simulink model "cal_hist_bin"  (R2015a)
settings: Solver=ode45  StartTime=0.0  StopTime=10.0  RelTol=1e-3
InitFcn:
  | %% DSPBuilder Start
  | alt_dspbuilder_update_model(bdroot)
  | %% DSPBuilder End
libraries: allblocks_alteradspbuilder2 x705
(part 1 of 9)
settings Model: Creator=ASUS  LastModifiedBy=ASUS

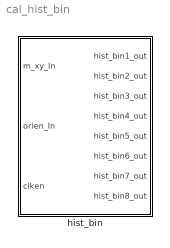
== system cal_hist_bin ==
  hist_bin : Subsystem

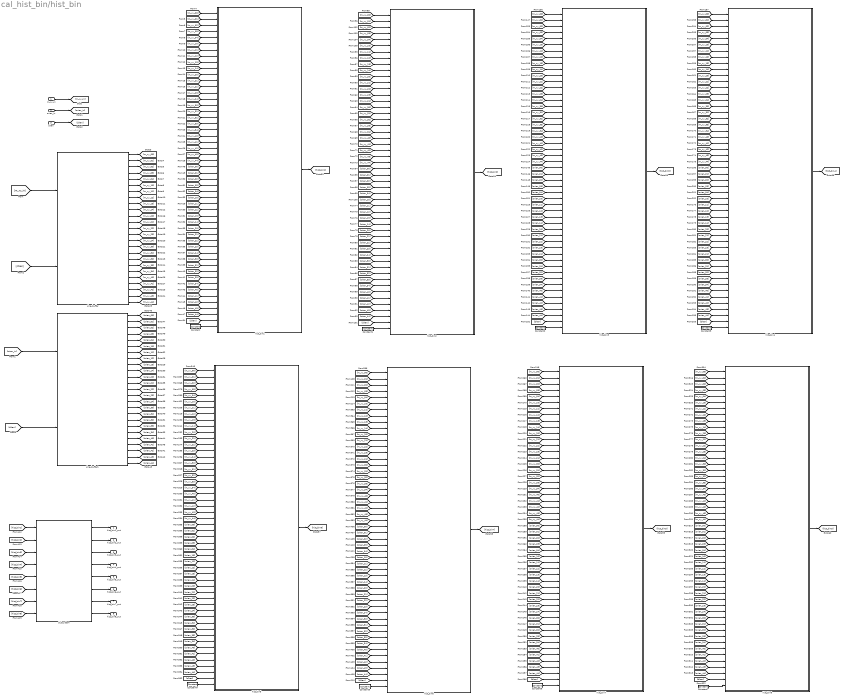
== system cal_hist_bin/hist_bin ==
  m_xy_In : Inport
  orien_In : Inport  Port=2
  clken : Inport  Port=3
  Constant : allblocks_alteradspbuilder2/Constant  mask_cst=1  BusType=Unsigned Integer  bwl=8  bwr=0  roundMode=Truncate  satMode=Wrap  SpecifyClock=off  allowFloatingPointOverride=on  logOutputs=off  logFile=C:\Users\ASUS\Desktop\sift_fpga_final\Octave_1\GradOrien\tb_Untitled1\Untitled1_hist%5Fbin_Constant.fixedpointlog
  Constant1 : allblocks_alteradspbuilder2/Constant  mask_cst=2  BusType=Unsigned Integer  bwl=8  bwr=0  roundMode=Truncate  satMode=Wrap  SpecifyClock=off  allowFloatingPointOverride=on  logOutputs=off  logFile=C:\Users\ASUS\Desktop\sift_fpga_final\Octave_1\GradOrien\tb_Untitled1\Untitled1_hist%5Fbin_Constant1.fixedpointlog
  Constant2 : allblocks_alteradspbuilder2/Constant  mask_cst=3  BusType=Unsigned Integer  bwl=8  bwr=0  roundMode=Truncate  satMode=Wrap  SpecifyClock=off  allowFloatingPointOverride=on  logOutputs=off  logFile=C:\Users\ASUS\Desktop\sift_fpga_final\Octave_1\GradOrien\tb_Untitled1\Untitled1_hist%5Fbin_Constant2.fixedpointlog
  Constant3 : allblocks_alteradspbuilder2/Constant  mask_cst=4  BusType=Unsigned Integer  bwl=8  bwr=0  roundMode=Truncate  satMode=Wrap  SpecifyClock=off  allowFloatingPointOverride=on  logOutputs=off  logFile=C:\Users\ASUS\Desktop\sift_fpga_final\Octave_1\GradOrien\tb_Untitled1\Untitled1_hist%5Fbin_Constant3.fixedpointlog
  Constant4 : allblocks_alteradspbuilder2/Constant  mask_cst=8  BusType=Unsigned Integer  bwl=8  bwr=0  roundMode=Truncate  satMode=Wrap  SpecifyClock=off  allowFloatingPointOverride=on  logOutputs=off  logFile=C:\Users\ASUS\Desktop\sift_fpga_final\Octave_1\GradOrien\tb_Untitled1\Untitled1_hist%5Fbin_Constant4.fixedpointlog
  Constant5 : allblocks_alteradspbuilder2/Constant  mask_cst=7  BusType=Unsigned Integer  bwl=8  bwr=0  roundMode=Truncate  satMode=Wrap  SpecifyClock=off  allowFloatingPointOverride=on  logOutputs=off  logFile=C:\Users\ASUS\Desktop\sift_fpga_final\Octave_1\GradOrien\tb_Untitled1\Untitled1_hist%5Fbin_Constant5.fixedpointlog
  Constant6 : allblocks_alteradspbuilder2/Constant  mask_cst=6  BusType=Unsigned Integer  bwl=8  bwr=0  roundMode=Truncate  satMode=Wrap  SpecifyClock=off  allowFloatingPointOverride=on  logOutputs=off  logFile=C:\Users\ASUS\Desktop\sift_fpga_final\Octave_1\GradOrien\tb_Untitled1\Untitled1_hist%5Fbin_Constant6.fixedpointlog
  Constant7 : allblocks_alteradspbuilder2/Constant  mask_cst=5  BusType=Unsigned Integer  bwl=8  bwr=0  roundMode=Truncate  satMode=Wrap  SpecifyClock=off  allowFloatingPointOverride=on  logOutputs=off  logFile=C:\Users\ASUS\Desktop\sift_fpga_final\Octave_1\GradOrien\tb_Untitled1\Untitled1_hist%5Fbin_Constant7.fixedpointlog
  Line_buffer : Subsystem
  Line_buffer1 : Subsystem
  Subsystem : Subsystem
  hist_bin1 : Subsystem
  hist_bin2 : Subsystem
  hist_bin3 : Subsystem
  hist_bin4 : Subsystem
  hist_bin5 : Subsystem
  hist_bin6 : Subsystem
  hist_bin7 : Subsystem
  hist_bin8 : Subsystem
  hist_bin1_out : Outport
  hist_bin2_out : Outport  Port=2
  hist_bin3_out : Outport  Port=3
  hist_bin4_out : Outport  Port=4
  hist_bin5_out : Outport  Port=5
  hist_bin6_out : Outport  Port=6
  hist_bin7_out : Outport  Port=7
  hist_bin8_out : Outport  Port=8
  wires:
  [hist_bin7] -> Subsystem/7(hist_in_bin7)
  [m_xy_in] -> Line_buffer/1(dataIn)
  [clken] -> Line_buffer/2(clken)
  [clken] -> Line_buffer1/2(clken)
  [orien_in] -> Line_buffer1/1(dataIn)
  clken/1 -> [clken]
  Line_buffer1/21(Out40) -> [orien_40]
  Line_buffer1/19(Out33) -> [orien_33]
  Line_buffer1/8(Out12) -> [orien_12]
  Line_buffer1/14(Out23) -> [orien_23]
  Line_buffer1/18(Out32) -> [orien_32]
  Line_buffer1/20(Out34) -> [orien_34]
  Line_buffer1/2(Out01) -> [orien_01]
  Line_buffer1/7(Out11) -> [orien_11]
  Line_buffer1/11(Out20) -> [orien_20]
  Line_buffer1/13(Out22) -> [orien_22]
  Line_buffer1/17(Out31) -> [orien_31]
  Line_buffer1/25(Out44) -> [orien_44]
  Line_buffer1/3(Out02) -> [orien_02]
  Line_buffer1/5(Out04) -> [orien_04]
  Line_buffer1/23(Out42) -> [orien_42]
  Line_buffer1/24(Out43) -> [orien_43]
  Line_buffer1/6(Out10) -> [orien_10]
  Line_buffer1/1(Out00) -> [orien_00]
  Line_buffer1/22(Out41) -> [orien_41]
  Line_buffer1/15(Out24) -> [orien_24]
  Line_buffer1/4(Out03) -> [orien_03]
  Line_buffer1/9(Out13) -> [orien_13]
  Line_buffer1/10(Out14) -> [orien_14]
  Line_buffer1/12(Out21) -> [orien_21]
  Line_buffer1/16(Out30) -> [orien_30]
  Line_buffer/24(Out43) -> [m_xy_43]
  Line_buffer/21(Out40) -> [m_xy_40]
  Line_buffer/23(Out42) -> [m_xy_42]
  Line_buffer/22(Out41) -> [m_xy_41]
  Line_buffer/25(Out44) -> [m_xy_44]
  Line_buffer/12(Out21) -> [m_xy_21]
  Line_buffer/15(Out24) -> [m_xy_24]
  Line_buffer/19(Out33) -> [m_xy_33]
  Line_buffer/18(Out32) -> [m_xy_32]
  Line_buffer/13(Out22) -> [m_xy_22]
  Line_buffer/11(Out20) -> [m_xy_20]
  Line_buffer/16(Out30) -> [m_xy_30]
  Line_buffer/14(Out23) -> [m_xy_23]
  Line_buffer/17(Out31) -> [m_xy_31]
  Line_buffer/20(Out34) -> [m_xy_34]
  [hist_bin1] -> Subsystem/1(hist_in_bin1)
  Line_buffer/1(Out00) -> [m_xy_00]
  [m_xy_04] -> hist_bin1/5(Mxy_In04)
  Line_buffer/2(Out01) -> [m_xy_01]
  hist_bin1/1(bin_out) -> [hist_bin1]
  [m_xy_10] -> hist_bin1/6(Mxy_In10)
  Line_buffer/9(Out13) -> [m_xy_13]
  [m_xy_13] -> hist_bin1/9(Mxy_In13)
  Line_buffer/10(Out14) -> [m_xy_14]
  Line_buffer/6(Out10) -> [m_xy_10]
  Line_buffer/7(Out11) -> [m_xy_11]
  [m_xy_11] -> hist_bin1/7(Mxy_In11)
  [m_xy_12] -> hist_bin1/8(Mxy_In12)
  Line_buffer/8(Out12) -> [m_xy_12]
  [m_xy_14] -> hist_bin1/10(Mxy_In14)
  [m_xy_22] -> hist_bin1/13(Mxy_In22)
  [m_xy_40] -> hist_bin1/21(Mxy_In40)
  [m_xy_43] -> hist_bin1/24(Mxy_In43)
  [m_xy_42] -> hist_bin1/23(Mxy_In42)
  [m_xy_44] -> hist_bin1/25(Mxy_In44)
  [m_xy_24] -> hist_bin1/15(Mxy_In24)
  [m_xy_21] -> hist_bin1/12(Mxy_In21)
  [m_xy_20] -> hist_bin1/11(Mxy_In20)
  [m_xy_23] -> hist_bin1/14(Mxy_In23)
  [m_xy_41] -> hist_bin1/22(Mxy_In41)
  [m_xy_01] -> hist_bin1/2(Mxy_In01)
  Line_buffer/4(Out03) -> [m_xy_03]
  Line_buffer/5(Out04) -> [m_xy_04]
  Line_buffer/3(Out02) -> [m_xy_02]
  [m_xy_31] -> hist_bin1/17(Mxy_In31)
  [m_xy_30] -> hist_bin1/16(Mxy_In30)
  [m_xy_34] -> hist_bin1/20(Mxy_In34)
  [m_xy_33] -> hist_bin1/19(Mxy_In33)
  [m_xy_32] -> hist_bin1/18(Mxy_In32)
  [m_xy_03] -> hist_bin1/4(Mxy_In03)
  [m_xy_02] -> hist_bin1/3(Mxy_In02)
  [hist_bin3] -> Subsystem/3(hist_in_bin3)
  [hist_bin4] -> Subsystem/4(hist_in_bin4)
  [orien_10] -> hist_bin1/31(Orien_In10)
  [orien_42] -> hist_bin1/48(Orien_In42)
  [orien_01] -> hist_bin1/27(Orien_In01)
  [orien_20] -> hist_bin1/36(Orien_In20)
  [orien_31] -> hist_bin1/42(Orien_In31)
  [orien_33] -> hist_bin1/44(Orien_In33)
  [orien_21] -> hist_bin1/37(Orien_In21)
  [orien_24] -> hist_bin1/40(Orien_In24)
  [orien_03] -> hist_bin1/29(Orien_In03)
  [orien_30] -> hist_bin1/41(Orien_In30)
  [orien_12] -> hist_bin1/33(Orien_In12)
  [orien_23] -> hist_bin1/39(Orien_In23)
  [orien_32] -> hist_bin1/43(Orien_In32)
  [orien_41] -> hist_bin1/47(Orien_In41)
  [orien_43] -> hist_bin1/49(Orien_In43)
  [orien_02] -> hist_bin1/28(Orien_In02)
  [orien_00] -> hist_bin1/26(Orien_In00)
  [orien_11] -> hist_bin1/32(Orien_In11)
  [orien_34] -> hist_bin1/45(Orien_In34)
  [orien_22] -> hist_bin1/38(Orien_In22)
  [orien_04] -> hist_bin1/30(Orien_In04)
  [orien_14] -> hist_bin1/35(Orien_In14)
  [orien_44] -> hist_bin1/50(Orien_In44)
  [orien_13] -> hist_bin1/34(Orien_In13)
  [orien_40] -> hist_bin1/46(Orien_In40)
  [clken] -> hist_bin1/51(clken)
  Constant/1 -> hist_bin1/52(bin_in)
  [m_xy_02] -> hist_bin2/3(Mxy_In02)
  [m_xy_04] -> hist_bin2/5(Mxy_In04)
  [m_xy_10] -> hist_bin2/6(Mxy_In10)
  [m_xy_23] -> hist_bin2/14(Mxy_In23)
  [m_xy_31] -> hist_bin2/17(Mxy_In31)
  [m_xy_30] -> hist_bin2/16(Mxy_In30)
  [m_xy_12] -> hist_bin2/8(Mxy_In12)
  [m_xy_32] -> hist_bin2/18(Mxy_In32)
  [m_xy_13] -> hist_bin2/9(Mxy_In13)
  [m_xy_33] -> hist_bin2/19(Mxy_In33)
  [m_xy_41] -> hist_bin2/22(Mxy_In41)
  [m_xy_01] -> hist_bin2/2(Mxy_In01)
  [m_xy_14] -> hist_bin2/10(Mxy_In14)
  [m_xy_40] -> hist_bin2/21(Mxy_In40)
  [m_xy_43] -> hist_bin2/24(Mxy_In43)
  [m_xy_20] -> hist_bin2/11(Mxy_In20)
  [m_xy_22] -> hist_bin2/13(Mxy_In22)
  [m_xy_24] -> hist_bin2/15(Mxy_In24)
  [m_xy_34] -> hist_bin2/20(Mxy_In34)
  [m_xy_03] -> hist_bin2/4(Mxy_In03)
  [m_xy_00] -> hist_bin2/1(Mxy_In00)
  [m_xy_11] -> hist_bin2/7(Mxy_In11)
  [m_xy_21] -> hist_bin2/12(Mxy_In21)
  [orien_31] -> hist_bin2/42(Orien_In31)
  [orien_34] -> hist_bin2/45(Orien_In34)
  [m_xy_42] -> hist_bin2/23(Mxy_In42)
  [orien_01] -> hist_bin2/27(Orien_In01)
  [orien_00] -> hist_bin2/26(Orien_In00)
  [orien_04] -> hist_bin2/30(Orien_In04)
  [orien_13] -> hist_bin2/34(Orien_In13)
  [orien_20] -> hist_bin2/36(Orien_In20)
  [orien_24] -> hist_bin2/40(Orien_In24)
  [orien_33] -> hist_bin2/44(Orien_In33)
  [orien_32] -> hist_bin2/43(Orien_In32)
  [orien_41] -> hist_bin2/47(Orien_In41)
  [orien_11] -> hist_bin2/32(Orien_In11)
  [orien_21] -> hist_bin2/37(Orien_In21)
  [orien_14] -> hist_bin2/35(Orien_In14)
  [orien_22] -> hist_bin2/38(Orien_In22)
  [orien_23] -> hist_bin2/39(Orien_In23)
  [orien_02] -> hist_bin2/28(Orien_In02)
  [orien_10] -> hist_bin2/31(Orien_In10)
  [orien_12] -> hist_bin2/33(Orien_In12)
  [orien_30] -> hist_bin2/41(Orien_In30)
  [m_xy_44] -> hist_bin2/25(Mxy_In44)
  [orien_03] -> hist_bin2/29(Orien_In03)
  [orien_40] -> hist_bin2/46(Orien_In40)
  [clken] -> hist_bin2/51(clken)
  hist_bin2/1(bin_out) -> [hist_bin2]
  [orien_42] -> hist_bin2/48(Orien_In42)
  [orien_44] -> hist_bin2/50(Orien_In44)
  [orien_43] -> hist_bin2/49(Orien_In43)
  Constant1/1 -> hist_bin2/52(bin_in)
  [m_xy_00] -> hist_bin1/1(Mxy_In00)
  Subsystem/4(bin4_out) -> hist_bin4_out/1
  Subsystem/3(bin3_out) -> hist_bin3_out/1
  [hist_bin8] -> Subsystem/8(hist_in_bin8)
  [hist_bin6] -> Subsystem/6(hist_in_bin6)
  [m_xy_01] -> hist_bin3/2(Mxy_In01)
  [m_xy_00] -> hist_bin3/1(Mxy_In00)
  [m_xy_03] -> hist_bin3/4(Mxy_In03)
  [m_xy_11] -> hist_bin3/7(Mxy_In11)
  [m_xy_13] -> hist_bin3/9(Mxy_In13)
  [m_xy_02] -> hist_bin3/3(Mxy_In02)
  [m_xy_34] -> hist_bin3/20(Mxy_In34)
  [m_xy_41] -> hist_bin3/22(Mxy_In41)
  [m_xy_40] -> hist_bin3/21(Mxy_In40)
  [m_xy_14] -> hist_bin3/10(Mxy_In14)
  [m_xy_43] -> hist_bin3/24(Mxy_In43)
  [m_xy_24] -> hist_bin3/15(Mxy_In24)
  [m_xy_42] -> hist_bin3/23(Mxy_In42)
  [m_xy_44] -> hist_bin3/25(Mxy_In44)
  [orien_01] -> hist_bin3/27(Orien_In01)
  [m_xy_30] -> hist_bin3/16(Mxy_In30)
  [orien_00] -> hist_bin3/26(Orien_In00)
  [m_xy_10] -> hist_bin3/6(Mxy_In10)
  [m_xy_21] -> hist_bin3/12(Mxy_In21)
  [m_xy_23] -> hist_bin3/14(Mxy_In23)
  [m_xy_31] -> hist_bin3/17(Mxy_In31)
  [m_xy_33] -> hist_bin3/19(Mxy_In33)
  [m_xy_22] -> hist_bin3/13(Mxy_In22)
  [m_xy_12] -> hist_bin3/8(Mxy_In12)
  [m_xy_32] -> hist_bin3/18(Mxy_In32)
  [m_xy_04] -> hist_bin3/5(Mxy_In04)
  [m_xy_20] -> hist_bin3/11(Mxy_In20)
  [orien_11] -> hist_bin3/32(Orien_In11)
  [orien_33] -> hist_bin3/44(Orien_In33)
  [orien_32] -> hist_bin3/43(Orien_In32)
  hist_bin3/1(bin_out) -> [hist_bin3]
  [orien_40] -> hist_bin3/46(Orien_In40)
  [orien_03] -> hist_bin3/29(Orien_In03)
  [orien_02] -> hist_bin3/28(Orien_In02)
  [orien_34] -> hist_bin3/45(Orien_In34)
  [orien_41] -> hist_bin3/47(Orien_In41)
  [orien_23] -> hist_bin3/39(Orien_In23)
  [orien_24] -> hist_bin3/40(Orien_In24)
  [orien_13] -> hist_bin3/34(Orien_In13)
  [orien_14] -> hist_bin3/35(Orien_In14)
  [orien_30] -> hist_bin3/41(Orien_In30)
  [orien_10] -> hist_bin3/31(Orien_In10)
  [orien_20] -> hist_bin3/36(Orien_In20)
  [orien_12] -> hist_bin3/33(Orien_In12)
  [orien_04] -> hist_bin3/30(Orien_In04)
  [orien_31] -> hist_bin3/42(Orien_In31)
  [orien_44] -> hist_bin3/50(Orien_In44)
  Constant2/1 -> hist_bin3/52(bin_in)
  [orien_22] -> hist_bin3/38(Orien_In22)
  [orien_43] -> hist_bin3/49(Orien_In43)
  [clken] -> hist_bin3/51(clken)
  [orien_42] -> hist_bin3/48(Orien_In42)
  [orien_21] -> hist_bin3/37(Orien_In21)
  [hist_bin5] -> Subsystem/5(hist_in_bin5)
  Subsystem/2(bin2_out) -> hist_bin2_out/1
  [m_xy_13] -> hist_bin5/9(Mxy_In13)
  [m_xy_03] -> hist_bin5/4(Mxy_In03)
  [m_xy_02] -> hist_bin5/3(Mxy_In02)
  [m_xy_12] -> hist_bin5/8(Mxy_In12)
  [m_xy_11] -> hist_bin5/7(Mxy_In11)
  [m_xy_14] -> hist_bin5/10(Mxy_In14)
  [m_xy_22] -> hist_bin5/13(Mxy_In22)
  [m_xy_31] -> hist_bin5/17(Mxy_In31)
  [m_xy_30] -> hist_bin5/16(Mxy_In30)
  [m_xy_33] -> hist_bin5/19(Mxy_In33)
  [m_xy_34] -> hist_bin5/20(Mxy_In34)
  [m_xy_04] -> hist_bin5/5(Mxy_In04)
  [m_xy_20] -> hist_bin5/11(Mxy_In20)
  [m_xy_41] -> hist_bin5/22(Mxy_In41)
  [m_xy_10] -> hist_bin5/6(Mxy_In10)
  [m_xy_24] -> hist_bin5/15(Mxy_In24)
  [m_xy_32] -> hist_bin5/18(Mxy_In32)
  [m_xy_01] -> hist_bin5/2(Mxy_In01)
  [m_xy_00] -> hist_bin5/1(Mxy_In00)
  [m_xy_21] -> hist_bin5/12(Mxy_In21)
  [m_xy_23] -> hist_bin5/14(Mxy_In23)
  [m_xy_41] -> hist_bin6/22(Mxy_In41)
  [orien_12] -> hist_bin5/33(Orien_In12)
  [orien_23] -> hist_bin5/39(Orien_In23)
  [orien_01] -> hist_bin5/27(Orien_In01)
  [m_xy_42] -> hist_bin5/23(Mxy_In42)
  [orien_03] -> hist_bin5/29(Orien_In03)
  [orien_11] -> hist_bin5/32(Orien_In11)
  [orien_34] -> hist_bin5/45(Orien_In34)
  [m_xy_11] -> hist_bin6/7(Mxy_In11)
  [m_xy_31] -> hist_bin6/17(Mxy_In31)
  [m_xy_44] -> hist_bin5/25(Mxy_In44)
  [orien_01] -> hist_bin6/27(Orien_In01)
  [orien_03] -> hist_bin6/29(Orien_In03)
  Constant4/1 -> hist_bin5/52(bin_in)
  [orien_41] -> hist_bin5/47(Orien_In41)
  [clken] -> hist_bin5/51(clken)
  [orien_32] -> hist_bin5/43(Orien_In32)
  [orien_04] -> hist_bin5/30(Orien_In04)
  [m_xy_00] -> hist_bin6/1(Mxy_In00)
  [m_xy_03] -> hist_bin6/4(Mxy_In03)
  [m_xy_40] -> hist_bin5/21(Mxy_In40)
  [m_xy_02] -> hist_bin6/3(Mxy_In02)
  [m_xy_04] -> hist_bin6/5(Mxy_In04)
  [m_xy_12] -> hist_bin6/8(Mxy_In12)
  [m_xy_20] -> hist_bin6/11(Mxy_In20)
  [m_xy_30] -> hist_bin6/16(Mxy_In30)
  [orien_13] -> hist_bin5/34(Orien_In13)
  [orien_33] -> hist_bin5/44(Orien_In33)
  [orien_40] -> hist_bin5/46(Orien_In40)
  [orien_24] -> hist_bin5/40(Orien_In24)
  [orien_02] -> hist_bin5/28(Orien_In02)
  [m_xy_14] -> hist_bin6/10(Mxy_In14)
  [m_xy_21] -> hist_bin6/12(Mxy_In21)
  [orien_44] -> hist_bin5/50(Orien_In44)
  [m_xy_23] -> hist_bin6/14(Mxy_In23)
  [orien_10] -> hist_bin5/31(Orien_In10)
  [orien_31] -> hist_bin5/42(Orien_In31)
  hist_bin5/1(bin_out) -> [hist_bin8]
  [m_xy_01] -> hist_bin6/2(Mxy_In01)
  [m_xy_33] -> hist_bin6/19(Mxy_In33)
  [m_xy_40] -> hist_bin6/21(Mxy_In40)
  [m_xy_43] -> hist_bin6/24(Mxy_In43)
  [m_xy_42] -> hist_bin6/23(Mxy_In42)
  [orien_00] -> hist_bin5/26(Orien_In00)
  [m_xy_44] -> hist_bin6/25(Mxy_In44)
  [orien_21] -> hist_bin5/37(Orien_In21)
  [orien_02] -> hist_bin6/28(Orien_In02)
  [m_xy_13] -> hist_bin6/9(Mxy_In13)
  [orien_04] -> hist_bin6/30(Orien_In04)
  [orien_11] -> hist_bin6/32(Orien_In11)
  [orien_43] -> hist_bin5/49(Orien_In43)
  [m_xy_22] -> hist_bin6/13(Mxy_In22)
  [orien_22] -> hist_bin5/38(Orien_In22)
  [orien_00] -> hist_bin6/26(Orien_In00)
  [orien_10] -> hist_bin6/31(Orien_In10)
  [orien_30] -> hist_bin5/41(Orien_In30)
  [m_xy_10] -> hist_bin6/6(Mxy_In10)
  [m_xy_32] -> hist_bin6/18(Mxy_In32)
  [m_xy_43] -> hist_bin5/24(Mxy_In43)
  [orien_14] -> hist_bin5/35(Orien_In14)
  [orien_20] -> hist_bin5/36(Orien_In20)
  [orien_42] -> hist_bin5/48(Orien_In42)
  [m_xy_24] -> hist_bin6/15(Mxy_In24)
  [m_xy_34] -> hist_bin6/20(Mxy_In34)
  hist_bin6/1(bin_out) -> [hist_bin7]
  [orien_02] -> hist_bin7/28(Orien_In02)
  [orien_30] -> hist_bin7/41(Orien_In30)
  [orien_33] -> hist_bin7/44(Orien_In33)
  [orien_42] -> hist_bin6/48(Orien_In42)
  [m_xy_20] -> hist_bin7/11(Mxy_In20)
  [orien_21] -> hist_bin7/37(Orien_In21)
  [orien_31] -> hist_bin7/42(Orien_In31)
  [orien_44] -> hist_bin6/50(Orien_In44)
  [m_xy_03] -> hist_bin7/4(Mxy_In03)
  [m_xy_21] -> hist_bin7/12(Mxy_In21)
  [m_xy_23] -> hist_bin7/14(Mxy_In23)
  [orien_22] -> hist_bin6/38(Orien_In22)
  [orien_31] -> hist_bin6/42(Orien_In31)
  [orien_40] -> hist_bin6/46(Orien_In40)
  [orien_43] -> hist_bin6/49(Orien_In43)
  [orien_34] -> hist_bin6/45(Orien_In34)
  [clken] -> hist_bin6/51(clken)
  [orien_41] -> hist_bin6/47(Orien_In41)
  [m_xy_00] -> hist_bin7/1(Mxy_In00)
  [m_xy_10] -> hist_bin7/6(Mxy_In10)
  [orien_30] -> hist_bin6/41(Orien_In30)
  [orien_13] -> hist_bin6/34(Orien_In13)
  [orien_24] -> hist_bin6/40(Orien_In24)
  [m_xy_13] -> hist_bin7/9(Mxy_In13)
  [m_xy_31] -> hist_bin7/17(Mxy_In31)
  [m_xy_40] -> hist_bin7/21(Mxy_In40)
  [m_xy_43] -> hist_bin7/24(Mxy_In43)
  Constant5/1 -> hist_bin6/52(bin_in)
  [m_xy_42] -> hist_bin7/23(Mxy_In42)
  [m_xy_24] -> hist_bin7/15(Mxy_In24)
  [m_xy_02] -> hist_bin7/3(Mxy_In02)
  [m_xy_44] -> hist_bin7/25(Mxy_In44)
  [m_xy_11] -> hist_bin7/7(Mxy_In11)
  [orien_14] -> hist_bin6/35(Orien_In14)
  [orien_32] -> hist_bin6/43(Orien_In32)
  [m_xy_33] -> hist_bin7/19(Mxy_In33)
  [orien_03] -> hist_bin7/29(Orien_In03)
  [orien_04] -> hist_bin7/30(Orien_In04)
  [orien_10] -> hist_bin7/31(Orien_In10)
  [orien_13] -> hist_bin7/34(Orien_In13)
  [orien_20] -> hist_bin6/36(Orien_In20)
  [m_xy_22] -> hist_bin7/13(Mxy_In22)
  [m_xy_34] -> hist_bin7/20(Mxy_In34)
  [orien_00] -> hist_bin7/26(Orien_In00)
  [m_xy_04] -> hist_bin7/5(Mxy_In04)
  [orien_23] -> hist_bin6/39(Orien_In23)
  [m_xy_41] -> hist_bin7/22(Mxy_In41)
  [orien_33] -> hist_bin6/44(Orien_In33)
  [orien_01] -> hist_bin7/27(Orien_In01)
  [orien_11] -> hist_bin7/32(Orien_In11)
  [m_xy_01] -> hist_bin7/2(Mxy_In01)
  [orien_21] -> hist_bin6/37(Orien_In21)
  [m_xy_14] -> hist_bin7/10(Mxy_In14)
  [m_xy_32] -> hist_bin7/18(Mxy_In32)
  [orien_12] -> hist_bin7/33(Orien_In12)
  [orien_12] -> hist_bin6/33(Orien_In12)
  [m_xy_30] -> hist_bin7/16(Mxy_In30)
  [orien_14] -> hist_bin7/35(Orien_In14)
  [orien_20] -> hist_bin7/36(Orien_In20)
  [orien_23] -> hist_bin7/39(Orien_In23)
  [orien_22] -> hist_bin7/38(Orien_In22)
  [m_xy_12] -> hist_bin7/8(Mxy_In12)
  [orien_24] -> hist_bin7/40(Orien_In24)
  [m_xy_42] -> hist_bin8/23(Mxy_In42)
  [orien_21] -> hist_bin8/37(Orien_In21)
  [orien_32] -> hist_bin8/43(Orien_In32)
  [orien_40] -> hist_bin7/46(Orien_In40)
  [m_xy_13] -> hist_bin8/9(Mxy_In13)
  [m_xy_44] -> hist_bin8/25(Mxy_In44)
  [orien_10] -> hist_bin8/31(Orien_In10)
  [m_xy_12] -> hist_bin8/8(Mxy_In12)
  [orien_20] -> hist_bin8/36(Orien_In20)
  [orien_23] -> hist_bin8/39(Orien_In23)
  [orien_30] -> hist_bin8/41(Orien_In30)
  [m_xy_30] -> hist_bin8/16(Mxy_In30)
  [m_xy_01] -> hist_bin8/2(Mxy_In01)
  [orien_43] -> hist_bin7/49(Orien_In43)
  hist_bin7/1(bin_out) -> [hist_bin5]
  [orien_41] -> hist_bin7/47(Orien_In41)
  [m_xy_02] -> hist_bin8/3(Mxy_In02)
  [orien_32] -> hist_bin7/43(Orien_In32)
  [m_xy_04] -> hist_bin8/5(Mxy_In04)
  [m_xy_11] -> hist_bin8/7(Mxy_In11)
  [m_xy_10] -> hist_bin8/6(Mxy_In10)
  [m_xy_14] -> hist_bin8/10(Mxy_In14)
  [m_xy_21] -> hist_bin8/12(Mxy_In21)
  [m_xy_33] -> hist_bin8/19(Mxy_In33)
  [m_xy_32] -> hist_bin8/18(Mxy_In32)
  [orien_42] -> hist_bin7/48(Orien_In42)
  [orien_34] -> hist_bin7/45(Orien_In34)
  [m_xy_34] -> hist_bin8/20(Mxy_In34)
  [m_xy_40] -> hist_bin8/21(Mxy_In40)
  [orien_00] -> hist_bin8/26(Orien_In00)
  [orien_03] -> hist_bin8/29(Orien_In03)
  [orien_04] -> hist_bin8/30(Orien_In04)
  Constant6/1 -> hist_bin7/52(bin_in)
  [m_xy_23] -> hist_bin8/14(Mxy_In23)
  [m_xy_03] -> hist_bin8/4(Mxy_In03)
  [orien_11] -> hist_bin8/32(Orien_In11)
  [m_xy_00] -> hist_bin8/1(Mxy_In00)
  [orien_13] -> hist_bin8/34(Orien_In13)
  [orien_12] -> hist_bin8/33(Orien_In12)
  [orien_24] -> hist_bin8/40(Orien_In24)
  [m_xy_24] -> hist_bin8/15(Mxy_In24)
  [orien_02] -> hist_bin8/28(Orien_In02)
  [orien_14] -> hist_bin8/35(Orien_In14)
  [orien_41] -> hist_bin8/47(Orien_In41)
  [orien_01] -> hist_bin8/27(Orien_In01)
  [m_xy_31] -> hist_bin8/17(Mxy_In31)
  [m_xy_41] -> hist_bin8/22(Mxy_In41)
  [orien_40] -> hist_bin8/46(Orien_In40)
  [orien_43] -> hist_bin8/49(Orien_In43)
  [orien_44] -> hist_bin7/50(Orien_In44)
  [orien_42] -> hist_bin8/48(Orien_In42)
  [m_xy_22] -> hist_bin8/13(Mxy_In22)
  [orien_34] -> hist_bin8/45(Orien_In34)
  [orien_44] -> hist_bin8/50(Orien_In44)
  [orien_22] -> hist_bin8/38(Orien_In22)
  [m_xy_20] -> hist_bin8/11(Mxy_In20)
  [clken] -> hist_bin8/51(clken)
  [clken] -> hist_bin7/51(clken)
  [orien_33] -> hist_bin8/44(Orien_In33)
  Constant7/1 -> hist_bin8/52(bin_in)
  [orien_31] -> hist_bin8/42(Orien_In31)
  hist_bin8/1(bin_out) -> [hist_bin5]
  [m_xy_43] -> hist_bin8/24(Mxy_In43)
  orien_In/1 -> [orien_in]
  [m_xy_01] -> hist_bin4/2(Mxy_In01)
  [m_xy_04] -> hist_bin4/5(Mxy_In04)
  [m_xy_12] -> hist_bin4/8(Mxy_In12)
  [m_xy_14] -> hist_bin4/10(Mxy_In14)
  [m_xy_21] -> hist_bin4/12(Mxy_In21)
  [m_xy_02] -> hist_bin4/3(Mxy_In02)
  [m_xy_23] -> hist_bin4/14(Mxy_In23)
  [m_xy_00] -> hist_bin4/1(Mxy_In00)
  [m_xy_13] -> hist_bin4/9(Mxy_In13)
  [m_xy_20] -> hist_bin4/11(Mxy_In20)
  [m_xy_11] -> hist_bin4/7(Mxy_In11)
  [m_xy_22] -> hist_bin4/13(Mxy_In22)
  [m_xy_24] -> hist_bin4/15(Mxy_In24)
  [m_xy_31] -> hist_bin4/17(Mxy_In31)
  [m_xy_10] -> hist_bin4/6(Mxy_In10)
  [m_xy_30] -> hist_bin4/16(Mxy_In30)
  [m_xy_33] -> hist_bin4/19(Mxy_In33)
  [m_xy_32] -> hist_bin4/18(Mxy_In32)
  [m_xy_34] -> hist_bin4/20(Mxy_In34)
  [m_xy_41] -> hist_bin4/22(Mxy_In41)
  [m_xy_40] -> hist_bin4/21(Mxy_In40)
  [m_xy_43] -> hist_bin4/24(Mxy_In43)
  [m_xy_03] -> hist_bin4/4(Mxy_In03)
  [m_xy_42] -> hist_bin4/23(Mxy_In42)
  [m_xy_44] -> hist_bin4/25(Mxy_In44)
  [orien_00] -> hist_bin4/26(Orien_In00)
  [orien_04] -> hist_bin4/30(Orien_In04)
  [orien_13] -> hist_bin4/34(Orien_In13)
  [orien_22] -> hist_bin4/38(Orien_In22)
  [orien_31] -> hist_bin4/42(Orien_In31)
  [orien_32] -> hist_bin4/43(Orien_In32)
  [orien_41] -> hist_bin4/47(Orien_In41)
  [orien_42] -> hist_bin4/48(Orien_In42)
  Constant3/1 -> hist_bin4/52(bin_in)
  [orien_11] -> hist_bin4/32(Orien_In11)
  [orien_12] -> hist_bin4/33(Orien_In12)
  [orien_44] -> hist_bin4/50(Orien_In44)
  [orien_14] -> hist_bin4/35(Orien_In14)
  [orien_33] -> hist_bin4/44(Orien_In33)
  [orien_03] -> hist_bin4/29(Orien_In03)
  [orien_40] -> hist_bin4/46(Orien_In40)
  hist_bin4/1(bin_out) -> [hist_bin4]
  [orien_21] -> hist_bin4/37(Orien_In21)
  [orien_10] -> hist_bin4/31(Orien_In10)
  [orien_01] -> hist_bin4/27(Orien_In01)
  [orien_02] -> hist_bin4/28(Orien_In02)
  [orien_20] -> hist_bin4/36(Orien_In20)
  [orien_30] -> hist_bin4/41(Orien_In30)
  [orien_34] -> hist_bin4/45(Orien_In34)
  [orien_43] -> hist_bin4/49(Orien_In43)
  [clken] -> hist_bin4/51(clken)
  [orien_24] -> hist_bin4/40(Orien_In24)
  [orien_23] -> hist_bin4/39(Orien_In23)
  m_xy_In/1 -> [m_xy_in]
  Subsystem/1(bin1_out) -> hist_bin1_out/1
  Subsystem/5(bin5_out) -> hist_bin5_out/1
  Subsystem/6(bin6_out) -> hist_bin6_out/1
  Subsystem/7(bin7_out) -> hist_bin7_out/1
  Subsystem/8(bin8_out) -> hist_bin8_out/1
  [hist_bin2] -> Subsystem/2(hist_in_bin2)

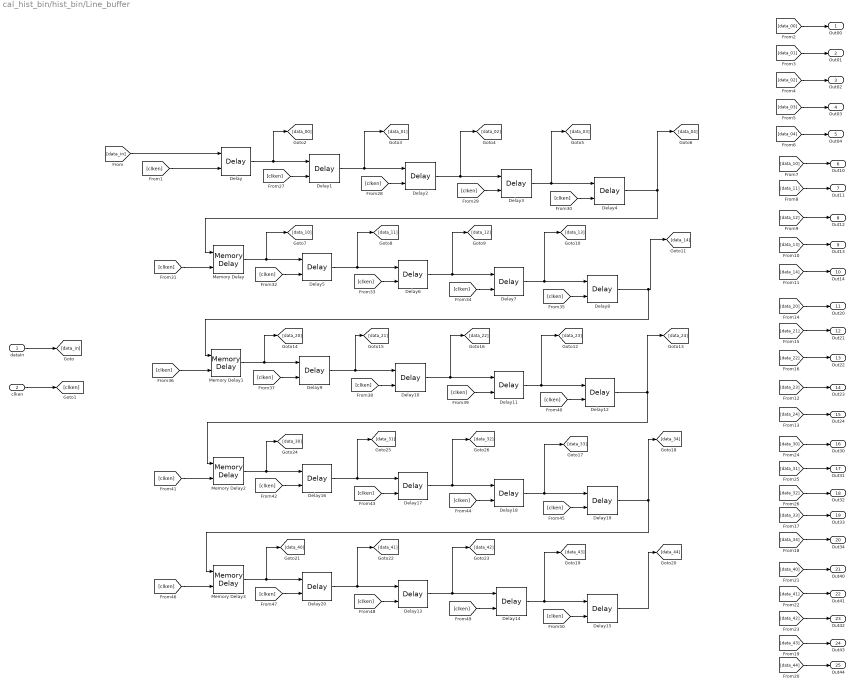
== system cal_hist_bin/hist_bin/Line_buffer ==
  dataIn : Inport
  clken : Inport  Port=2
  Delay : allblocks_alteradspbuilder2/Delay  pipeline=1  pipeline_display=1  ClockPhase=1  use_ena=on  use_sclr=off  allowFloatingPointOverride=on  logOutputs=off  logFile=C:\Users\ASUS\Desktop\sift_fpga_final\Octave_1\GradOrien\tb_Untitled1\Untitled1_hist%5Fbin_Line%5Fbuffer_Delay.fixedpointlog  use_init=off  reset_value=1
  Delay1 : allblocks_alteradspbuilder2/Delay  pipeline=1  pipeline_display=1  ClockPhase=1  use_ena=on  use_sclr=off  allowFloatingPointOverride=on  logOutputs=off  logFile=C:\Users\ASUS\Desktop\sift_fpga_final\Octave_1\GradOrien\tb_Untitled1\Untitled1_hist%5Fbin_Line%5Fbuffer_Delay1.fixedpointlog  use_init=off  reset_value=1
  Delay10 : allblocks_alteradspbuilder2/Delay  pipeline=1  pipeline_display=1  ClockPhase=1  use_ena=on  use_sclr=off  allowFloatingPointOverride=on  logOutputs=off  logFile=C:\Users\ASUS\Desktop\sift_fpga_final\Octave_1\GradOrien\tb_Untitled1\Untitled1_hist%5Fbin_Line%5Fbuffer_Delay10.fixedpointlog  use_init=off  reset_value=1
  Delay11 : allblocks_alteradspbuilder2/Delay  pipeline=1  pipeline_display=1  ClockPhase=1  use_ena=on  use_sclr=off  allowFloatingPointOverride=on  logOutputs=off  logFile=C:\Users\ASUS\Desktop\sift_fpga_final\Octave_1\GradOrien\tb_Untitled1\Untitled1_hist%5Fbin_Line%5Fbuffer_Delay11.fixedpointlog  use_init=off  reset_value=1
  Delay12 : allblocks_alteradspbuilder2/Delay  pipeline=1  pipeline_display=1  ClockPhase=1  use_ena=on  use_sclr=off  allowFloatingPointOverride=on  logOutputs=off  logFile=C:\Users\ASUS\Desktop\sift_fpga_final\Octave_1\GradOrien\tb_Untitled1\Untitled1_hist%5Fbin_Line%5Fbuffer_Delay12.fixedpointlog  use_init=off  reset_value=1
  Delay13 : allblocks_alteradspbuilder2/Delay  pipeline=1  pipeline_display=1  ClockPhase=1  use_ena=on  use_sclr=off  allowFloatingPointOverride=on  logOutputs=off  logFile=C:\Users\ASUS\Desktop\sift_fpga_final\Octave_1\GradOrien\tb_Untitled1\Untitled1_hist%5Fbin_Line%5Fbuffer_Delay13.fixedpointlog  use_init=off  reset_value=1
  Delay14 : allblocks_alteradspbuilder2/Delay  pipeline=1  pipeline_display=1  ClockPhase=1  use_ena=on  use_sclr=off  allowFloatingPointOverride=on  logOutputs=off  logFile=C:\Users\ASUS\Desktop\sift_fpga_final\Octave_1\GradOrien\tb_Untitled1\Untitled1_hist%5Fbin_Line%5Fbuffer_Delay14.fixedpointlog  use_init=off  reset_value=1
  Delay15 : allblocks_alteradspbuilder2/Delay  pipeline=1  pipeline_display=1  ClockPhase=1  use_ena=on  use_sclr=off  allowFloatingPointOverride=on  logOutputs=off  logFile=C:\Users\ASUS\Desktop\sift_fpga_final\Octave_1\GradOrien\tb_Untitled1\Untitled1_hist%5Fbin_Line%5Fbuffer_Delay15.fixedpointlog  use_init=off  reset_value=1
  Delay16 : allblocks_alteradspbuilder2/Delay  pipeline=1  pipeline_display=1  ClockPhase=1  use_ena=on  use_sclr=off  allowFloatingPointOverride=on  logOutputs=off  logFile=C:\Users\ASUS\Desktop\sift_fpga_final\Octave_1\GradOrien\tb_Untitled1\Untitled1_hist%5Fbin_Line%5Fbuffer_Delay16.fixedpointlog  use_init=off  reset_value=1
  Delay17 : allblocks_alteradspbuilder2/Delay  pipeline=1  pipeline_display=1  ClockPhase=1  use_ena=on  use_sclr=off  allowFloatingPointOverride=on  logOutputs=off  logFile=C:\Users\ASUS\Desktop\sift_fpga_final\Octave_1\GradOrien\tb_Untitled1\Untitled1_hist%5Fbin_Line%5Fbuffer_Delay17.fixedpointlog  use_init=off  reset_value=1
  Delay18 : allblocks_alteradspbuilder2/Delay  pipeline=1  pipeline_display=1  ClockPhase=1  use_ena=on  use_sclr=off  allowFloatingPointOverride=on  logOutputs=off  logFile=C:\Users\ASUS\Desktop\sift_fpga_final\Octave_1\GradOrien\tb_Untitled1\Untitled1_hist%5Fbin_Line%5Fbuffer_Delay18.fixedpointlog  use_init=off  reset_value=1
  Delay19 : allblocks_alteradspbuilder2/Delay  pipeline=1  pipeline_display=1  ClockPhase=1  use_ena=on  use_sclr=off  allowFloatingPointOverride=on  logOutputs=off  logFile=C:\Users\ASUS\Desktop\sift_fpga_final\Octave_1\GradOrien\tb_Untitled1\Untitled1_hist%5Fbin_Line%5Fbuffer_Delay19.fixedpointlog  use_init=off  reset_value=1
  Delay2 : allblocks_alteradspbuilder2/Delay  pipeline=1  pipeline_display=1  ClockPhase=1  use_ena=on  use_sclr=off  allowFloatingPointOverride=on  logOutputs=off  logFile=C:\Users\ASUS\Desktop\sift_fpga_final\Octave_1\GradOrien\tb_Untitled1\Untitled1_hist%5Fbin_Line%5Fbuffer_Delay2.fixedpointlog  use_init=off  reset_value=1
  Delay20 : allblocks_alteradspbuilder2/Delay  pipeline=1  pipeline_display=1  ClockPhase=1  use_ena=on  use_sclr=off  allowFloatingPointOverride=on  logOutputs=off  logFile=C:\Users\ASUS\Desktop\sift_fpga_final\Octave_1\GradOrien\tb_Untitled1\Untitled1_hist%5Fbin_Line%5Fbuffer_Delay20.fixedpointlog  use_init=off  reset_value=1
  Delay3 : allblocks_alteradspbuilder2/Delay  pipeline=1  pipeline_display=1  ClockPhase=1  use_ena=on  use_sclr=off  allowFloatingPointOverride=on  logOutputs=off  logFile=C:\Users\ASUS\Desktop\sift_fpga_final\Octave_1\GradOrien\tb_Untitled1\Untitled1_hist%5Fbin_Line%5Fbuffer_Delay3.fixedpointlog  use_init=off  reset_value=1
  Delay4 : allblocks_alteradspbuilder2/Delay  pipeline=1  pipeline_display=1  ClockPhase=1  use_ena=on  use_sclr=off  allowFloatingPointOverride=on  logOutputs=off  logFile=C:\Users\ASUS\Desktop\sift_fpga_final\Octave_1\GradOrien\tb_Untitled1\Untitled1_hist%5Fbin_Line%5Fbuffer_Delay4.fixedpointlog  use_init=off  reset_value=1
  Delay5 : allblocks_alteradspbuilder2/Delay  pipeline=1  pipeline_display=1  ClockPhase=1  use_ena=on  use_sclr=off  allowFloatingPointOverride=on  logOutputs=off  logFile=C:\Users\ASUS\Desktop\sift_fpga_final\Octave_1\GradOrien\tb_Untitled1\Untitled1_hist%5Fbin_Line%5Fbuffer_Delay5.fixedpointlog  use_init=off  reset_value=1
  Delay6 : allblocks_alteradspbuilder2/Delay  pipeline=1  pipeline_display=1  ClockPhase=1  use_ena=on  use_sclr=off  allowFloatingPointOverride=on  logOutputs=off  logFile=C:\Users\ASUS\Desktop\sift_fpga_final\Octave_1\GradOrien\tb_Untitled1\Untitled1_hist%5Fbin_Line%5Fbuffer_Delay6.fixedpointlog  use_init=off  reset_value=1
  Delay7 : allblocks_alteradspbuilder2/Delay  pipeline=1  pipeline_display=1  ClockPhase=1  use_ena=on  use_sclr=off  allowFloatingPointOverride=on  logOutputs=off  logFile=C:\Users\ASUS\Desktop\sift_fpga_final\Octave_1\GradOrien\tb_Untitled1\Untitled1_hist%5Fbin_Line%5Fbuffer_Delay7.fixedpointlog  use_init=off  reset_value=1
  Delay8 : allblocks_alteradspbuilder2/Delay  pipeline=1  pipeline_display=1  ClockPhase=1  use_ena=on  use_sclr=off  allowFloatingPointOverride=on  logOutputs=off  logFile=C:\Users\ASUS\Desktop\sift_fpga_final\Octave_1\GradOrien\tb_Untitled1\Untitled1_hist%5Fbin_Line%5Fbuffer_Delay8.fixedpointlog  use_init=off  reset_value=1
  Delay9 : allblocks_alteradspbuilder2/Delay  pipeline=1  pipeline_display=1  ClockPhase=1  use_ena=on  use_sclr=off  allowFloatingPointOverride=on  logOutputs=off  logFile=C:\Users\ASUS\Desktop\sift_fpga_final\Octave_1\GradOrien\tb_Untitled1\Untitled1_hist%5Fbin_Line%5Fbuffer_Delay9.fixedpointlog  use_init=off  reset_value=1
  Memory Delay : allblocks_alteradspbuilder2/Memory Delay  BusType=Unsigned Integer  bwl=8  bwr=0  pipeline=640  pipeline_display=640  ram_type=AUTO  use_ena=on  use_sclr=off  allowFloatingPointOverride=on  logOutputs=off  logFile=C:\Users\ASUS\Desktop\sift_fpga_final\Octave_1\GradOrien\tb_Untitled1\Untitled1_hist%5Fbin_Line%5Fbuffer_Memory+Delay.fixedpointlog
  Memory Delay1 : allblocks_alteradspbuilder2/Memory Delay  BusType=Unsigned Integer  bwl=8  bwr=0  pipeline=640  pipeline_display=640  ram_type=AUTO  use_ena=on  use_sclr=off  allowFloatingPointOverride=on  logOutputs=off  logFile=C:\Users\ASUS\Desktop\sift_fpga_final\Octave_1\GradOrien\tb_Untitled1\Untitled1_hist%5Fbin_Line%5Fbuffer_Memory+Delay1.fixedpointlog
  Memory Delay2 : allblocks_alteradspbuilder2/Memory Delay  BusType=Unsigned Integer  bwl=8  bwr=0  pipeline=640  pipeline_display=640  ram_type=AUTO  use_ena=on  use_sclr=off  allowFloatingPointOverride=on  logOutputs=off  logFile=C:\Users\ASUS\Desktop\sift_fpga_final\Octave_1\GradOrien\tb_Untitled1\Untitled1_hist%5Fbin_Line%5Fbuffer_Memory+Delay2.fixedpointlog
  Memory Delay3 : allblocks_alteradspbuilder2/Memory Delay  BusType=Unsigned Integer  bwl=8  bwr=0  pipeline=640  pipeline_display=640  ram_type=AUTO  use_ena=on  use_sclr=off  allowFloatingPointOverride=on  logOutputs=off  logFile=C:\Users\ASUS\Desktop\sift_fpga_final\Octave_1\GradOrien\tb_Untitled1\Untitled1_hist%5Fbin_Line%5Fbuffer_Memory+Delay3.fixedpointlog
  Out00 : Outport
  Out01 : Outport  Port=2
  Out02 : Outport  Port=3
  Out03 : Outport  Port=4
  Out04 : Outport  Port=5
  Out10 : Outport  Port=6
  Out11 : Outport  Port=7
  Out12 : Outport  Port=8
  Out13 : Outport  Port=9
  Out14 : Outport  Port=10
  Out20 : Outport  Port=11
  Out21 : Outport  Port=12
  Out22 : Outport  Port=13
  Out23 : Outport  Port=14
  Out24 : Outport  Port=15
  Out30 : Outport  Port=16
  Out31 : Outport  Port=17
  Out32 : Outport  Port=18
  Out33 : Outport  Port=19
  Out34 : Outport  Port=20
  Out40 : Outport  Port=21
  Out41 : Outport  Port=22
  Out42 : Outport  Port=23
  Out43 : Outport  Port=24
  Out44 : Outport  Port=25
  wires:
  [clken] -> Delay11/2
  Delay11/1 -> [data_23], Delay12/1
  [clken] -> Delay12/2
  [clken] -> Delay10/2
  Delay8/1 -> Memory Delay1/1, [data_14]
  [clken] -> Memory Delay1/2
  Delay9/1 -> [data_21], Delay10/1
  Memory Delay1/1 -> [data_20], Delay9/1
  Delay10/1 -> [data_22], Delay11/1
  [clken] -> Delay9/2
  [clken] -> Delay4/2
  [data_03] -> Out03/1
  [data_04] -> Out04/1
  [data_02] -> Out02/1
  Delay/1 -> [data_00], Delay1/1
  [data_32] -> Out32/1
  [data_44] -> Out44/1
  [data_31] -> Out31/1
  [data_40] -> Out40/1
  [data_34] -> Out34/1
  [data_30] -> Out30/1
  [data_33] -> Out33/1
  [data_43] -> Out43/1
  [data_42] -> Out42/1
  [data_41] -> Out41/1
  [clken] -> Delay1/2
  [clken] -> Delay/2
  [data_in] -> Delay/1
  [clken] -> Delay2/2
  Delay2/1 -> [data_02], Delay3/1
  Delay1/1 -> [data_01], Delay2/1
  [clken] -> Delay3/2
  [data_01] -> Out01/1
  clken/1 -> [clken]
  [data_00] -> Out00/1
  [data_21] -> Out21/1
  [data_20] -> Out20/1
  [data_23] -> Out23/1
  [data_22] -> Out22/1
  [data_24] -> Out24/1
  dataIn/1 -> [data_in]
  [data_10] -> Out10/1
  [data_11] -> Out11/1
  [data_12] -> Out12/1
  [data_13] -> Out13/1
  [data_14] -> Out14/1
  Delay4/1 -> Memory Delay/1, [data_04]
  [clken] -> Memory Delay/2
  Delay12/1 -> [data_24], Memory Delay2/1
  [clken] -> Memory Delay2/2
  Memory Delay2/1 -> [data_30], Delay16/1
  [clken] -> Delay16/2
  [clken] -> Delay14/2
  [clken] -> Delay15/2
  [clken] -> Memory Delay3/2
  Delay17/1 -> [data_32], Delay18/1
  Delay18/1 -> [data_33], Delay19/1
  Memory Delay3/1 -> [data_40], Delay20/1
  [clken] -> Delay20/2
  [clken] -> Delay19/2
  Delay13/1 -> [data_42], Delay14/1
  Delay19/1 -> Memory Delay3/1, [data_34]
  Delay14/1 -> [data_43], Delay15/1
  Delay15/1 -> [data_44]
  [clken] -> Delay17/2
  [clken] -> Delay18/2
  [clken] -> Delay13/2
  Delay16/1 -> [data_31], Delay17/1
  Delay20/1 -> [data_41], Delay13/1
  Memory Delay/1 -> [data_10], Delay5/1
  [clken] -> Delay7/2
  [clken] -> Delay6/2
  Delay5/1 -> [data_11], Delay6/1
  [clken] -> Delay8/2
  [clken] -> Delay5/2
  Delay7/1 -> [data_13], Delay8/1
  Delay6/1 -> [data_12], Delay7/1
  Delay3/1 -> [data_03], Delay4/1

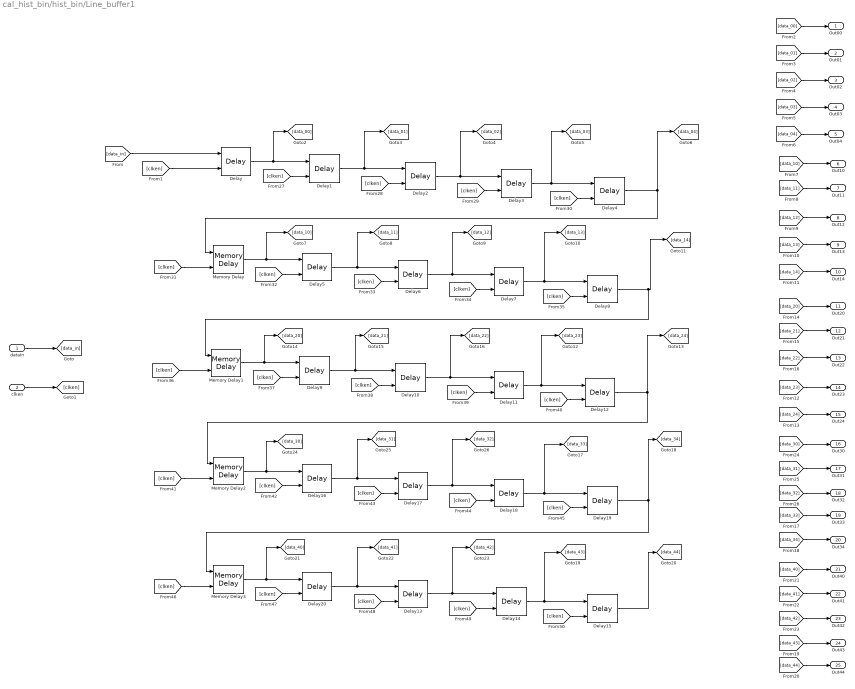
== system cal_hist_bin/hist_bin/Line_buffer1 ==
  dataIn : Inport
  clken : Inport  Port=2
  Delay : allblocks_alteradspbuilder2/Delay  pipeline=1  pipeline_display=1  ClockPhase=1  use_ena=on  use_sclr=off  allowFloatingPointOverride=on  logOutputs=off  logFile=C:\Users\ASUS\Desktop\sift_fpga_final\Octave_1\GradOrien\tb_Untitled1\Untitled1_hist%5Fbin_Line%5Fbuffer1_Delay.fixedpointlog  use_init=off  reset_value=1
  Delay1 : allblocks_alteradspbuilder2/Delay  pipeline=1  pipeline_display=1  ClockPhase=1  use_ena=on  use_sclr=off  allowFloatingPointOverride=on  logOutputs=off  logFile=C:\Users\ASUS\Desktop\sift_fpga_final\Octave_1\GradOrien\tb_Untitled1\Untitled1_hist%5Fbin_Line%5Fbuffer1_Delay1.fixedpointlog  use_init=off  reset_value=1
  Delay10 : allblocks_alteradspbuilder2/Delay  pipeline=1  pipeline_display=1  ClockPhase=1  use_ena=on  use_sclr=off  allowFloatingPointOverride=on  logOutputs=off  logFile=C:\Users\ASUS\Desktop\sift_fpga_final\Octave_1\GradOrien\tb_Untitled1\Untitled1_hist%5Fbin_Line%5Fbuffer1_Delay10.fixedpointlog  use_init=off  reset_value=1
  Delay11 : allblocks_alteradspbuilder2/Delay  pipeline=1  pipeline_display=1  ClockPhase=1  use_ena=on  use_sclr=off  allowFloatingPointOverride=on  logOutputs=off  logFile=C:\Users\ASUS\Desktop\sift_fpga_final\Octave_1\GradOrien\tb_Untitled1\Untitled1_hist%5Fbin_Line%5Fbuffer1_Delay11.fixedpointlog  use_init=off  reset_value=1
  Delay12 : allblocks_alteradspbuilder2/Delay  pipeline=1  pipeline_display=1  ClockPhase=1  use_ena=on  use_sclr=off  allowFloatingPointOverride=on  logOutputs=off  logFile=C:\Users\ASUS\Desktop\sift_fpga_final\Octave_1\GradOrien\tb_Untitled1\Untitled1_hist%5Fbin_Line%5Fbuffer1_Delay12.fixedpointlog  use_init=off  reset_value=1
  Delay13 : allblocks_alteradspbuilder2/Delay  pipeline=1  pipeline_display=1  ClockPhase=1  use_ena=on  use_sclr=off  allowFloatingPointOverride=on  logOutputs=off  logFile=C:\Users\ASUS\Desktop\sift_fpga_final\Octave_1\GradOrien\tb_Untitled1\Untitled1_hist%5Fbin_Line%5Fbuffer1_Delay13.fixedpointlog  use_init=off  reset_value=1
  Delay14 : allblocks_alteradspbuilder2/Delay  pipeline=1  pipeline_display=1  ClockPhase=1  use_ena=on  use_sclr=off  allowFloatingPointOverride=on  logOutputs=off  logFile=C:\Users\ASUS\Desktop\sift_fpga_final\Octave_1\GradOrien\tb_Untitled1\Untitled1_hist%5Fbin_Line%5Fbuffer1_Delay14.fixedpointlog  use_init=off  reset_value=1
  Delay15 : allblocks_alteradspbuilder2/Delay  pipeline=1  pipeline_display=1  ClockPhase=1  use_ena=on  use_sclr=off  allowFloatingPointOverride=on  logOutputs=off  logFile=C:\Users\ASUS\Desktop\sift_fpga_final\Octave_1\GradOrien\tb_Untitled1\Untitled1_hist%5Fbin_Line%5Fbuffer1_Delay15.fixedpointlog  use_init=off  reset_value=1
  Delay16 : allblocks_alteradspbuilder2/Delay  pipeline=1  pipeline_display=1  ClockPhase=1  use_ena=on  use_sclr=off  allowFloatingPointOverride=on  logOutputs=off  logFile=C:\Users\ASUS\Desktop\sift_fpga_final\Octave_1\GradOrien\tb_Untitled1\Untitled1_hist%5Fbin_Line%5Fbuffer1_Delay16.fixedpointlog  use_init=off  reset_value=1
  Delay17 : allblocks_alteradspbuilder2/Delay  pipeline=1  pipeline_display=1  ClockPhase=1  use_ena=on  use_sclr=off  allowFloatingPointOverride=on  logOutputs=off  logFile=C:\Users\ASUS\Desktop\sift_fpga_final\Octave_1\GradOrien\tb_Untitled1\Untitled1_hist%5Fbin_Line%5Fbuffer1_Delay17.fixedpointlog  use_init=off  reset_value=1
  Delay18 : allblocks_alteradspbuilder2/Delay  pipeline=1  pipeline_display=1  ClockPhase=1  use_ena=on  use_sclr=off  allowFloatingPointOverride=on  logOutputs=off  logFile=C:\Users\ASUS\Desktop\sift_fpga_final\Octave_1\GradOrien\tb_Untitled1\Untitled1_hist%5Fbin_Line%5Fbuffer1_Delay18.fixedpointlog  use_init=off  reset_value=1
  Delay19 : allblocks_alteradspbuilder2/Delay  pipeline=1  pipeline_display=1  ClockPhase=1  use_ena=on  use_sclr=off  allowFloatingPointOverride=on  logOutputs=off  logFile=C:\Users\ASUS\Desktop\sift_fpga_final\Octave_1\GradOrien\tb_Untitled1\Untitled1_hist%5Fbin_Line%5Fbuffer1_Delay19.fixedpointlog  use_init=off  reset_value=1
  Delay2 : allblocks_alteradspbuilder2/Delay  pipeline=1  pipeline_display=1  ClockPhase=1  use_ena=on  use_sclr=off  allowFloatingPointOverride=on  logOutputs=off  logFile=C:\Users\ASUS\Desktop\sift_fpga_final\Octave_1\GradOrien\tb_Untitled1\Untitled1_hist%5Fbin_Line%5Fbuffer1_Delay2.fixedpointlog  use_init=off  reset_value=1
  Delay20 : allblocks_alteradspbuilder2/Delay  pipeline=1  pipeline_display=1  ClockPhase=1  use_ena=on  use_sclr=off  allowFloatingPointOverride=on  logOutputs=off  logFile=C:\Users\ASUS\Desktop\sift_fpga_final\Octave_1\GradOrien\tb_Untitled1\Untitled1_hist%5Fbin_Line%5Fbuffer1_Delay20.fixedpointlog  use_init=off  reset_value=1
  Delay3 : allblocks_alteradspbuilder2/Delay  pipeline=1  pipeline_display=1  ClockPhase=1  use_ena=on  use_sclr=off  allowFloatingPointOverride=on  logOutputs=off  logFile=C:\Users\ASUS\Desktop\sift_fpga_final\Octave_1\GradOrien\tb_Untitled1\Untitled1_hist%5Fbin_Line%5Fbuffer1_Delay3.fixedpointlog  use_init=off  reset_value=1
  Delay4 : allblocks_alteradspbuilder2/Delay  pipeline=1  pipeline_display=1  ClockPhase=1  use_ena=on  use_sclr=off  allowFloatingPointOverride=on  logOutputs=off  logFile=C:\Users\ASUS\Desktop\sift_fpga_final\Octave_1\GradOrien\tb_Untitled1\Untitled1_hist%5Fbin_Line%5Fbuffer1_Delay4.fixedpointlog  use_init=off  reset_value=1
  Delay5 : allblocks_alteradspbuilder2/Delay  pipeline=1  pipeline_display=1  ClockPhase=1  use_ena=on  use_sclr=off  allowFloatingPointOverride=on  logOutputs=off  logFile=C:\Users\ASUS\Desktop\sift_fpga_final\Octave_1\GradOrien\tb_Untitled1\Untitled1_hist%5Fbin_Line%5Fbuffer1_Delay5.fixedpointlog  use_init=off  reset_value=1
  Delay6 : allblocks_alteradspbuilder2/Delay  pipeline=1  pipeline_display=1  ClockPhase=1  use_ena=on  use_sclr=off  allowFloatingPointOverride=on  logOutputs=off  logFile=C:\Users\ASUS\Desktop\sift_fpga_final\Octave_1\GradOrien\tb_Untitled1\Untitled1_hist%5Fbin_Line%5Fbuffer1_Delay6.fixedpointlog  use_init=off  reset_value=1
  Delay7 : allblocks_alteradspbuilder2/Delay  pipeline=1  pipeline_display=1  ClockPhase=1  use_ena=on  use_sclr=off  allowFloatingPointOverride=on  logOutputs=off  logFile=C:\Users\ASUS\Desktop\sift_fpga_final\Octave_1\GradOrien\tb_Untitled1\Untitled1_hist%5Fbin_Line%5Fbuffer1_Delay7.fixedpointlog  use_init=off  reset_value=1
  Delay8 : allblocks_alteradspbuilder2/Delay  pipeline=1  pipeline_display=1  ClockPhase=1  use_ena=on  use_sclr=off  allowFloatingPointOverride=on  logOutputs=off  logFile=C:\Users\ASUS\Desktop\sift_fpga_final\Octave_1\GradOrien\tb_Untitled1\Untitled1_hist%5Fbin_Line%5Fbuffer1_Delay8.fixedpointlog  use_init=off  reset_value=1
  Delay9 : allblocks_alteradspbuilder2/Delay  pipeline=1  pipeline_display=1  ClockPhase=1  use_ena=on  use_sclr=off  allowFloatingPointOverride=on  logOutputs=off  logFile=C:\Users\ASUS\Desktop\sift_fpga_final\Octave_1\GradOrien\tb_Untitled1\Untitled1_hist%5Fbin_Line%5Fbuffer1_Delay9.fixedpointlog  use_init=off  reset_value=1
  Memory Delay : allblocks_alteradspbuilder2/Memory Delay  BusType=Unsigned Integer  bwl=8  bwr=0  pipeline=640  pipeline_display=640  ram_type=AUTO  use_ena=on  use_sclr=off  allowFloatingPointOverride=on  logOutputs=off  logFile=C:\Users\ASUS\Desktop\sift_fpga_final\Octave_1\GradOrien\tb_Untitled1\Untitled1_hist%5Fbin_Line%5Fbuffer1_Memory+Delay.fixedpointlog
  Memory Delay1 : allblocks_alteradspbuilder2/Memory Delay  BusType=Unsigned Integer  bwl=8  bwr=0  pipeline=640  pipeline_display=640  ram_type=AUTO  use_ena=on  use_sclr=off  allowFloatingPointOverride=on  logOutputs=off  logFile=C:\Users\ASUS\Desktop\sift_fpga_final\Octave_1\GradOrien\tb_Untitled1\Untitled1_hist%5Fbin_Line%5Fbuffer1_Memory+Delay1.fixedpointlog
  Memory Delay2 : allblocks_alteradspbuilder2/Memory Delay  BusType=Unsigned Integer  bwl=8  bwr=0  pipeline=640  pipeline_display=640  ram_type=AUTO  use_ena=on  use_sclr=off  allowFloatingPointOverride=on  logOutputs=off  logFile=C:\Users\ASUS\Desktop\sift_fpga_final\Octave_1\GradOrien\tb_Untitled1\Untitled1_hist%5Fbin_Line%5Fbuffer1_Memory+Delay2.fixedpointlog
  Memory Delay3 : allblocks_alteradspbuilder2/Memory Delay  BusType=Unsigned Integer  bwl=8  bwr=0  pipeline=640  pipeline_display=640  ram_type=AUTO  use_ena=on  use_sclr=off  allowFloatingPointOverride=on  logOutputs=off  logFile=C:\Users\ASUS\Desktop\sift_fpga_final\Octave_1\GradOrien\tb_Untitled1\Untitled1_hist%5Fbin_Line%5Fbuffer1_Memory+Delay3.fixedpointlog
  Out00 : Outport
  Out01 : Outport  Port=2
  Out02 : Outport  Port=3
  Out03 : Outport  Port=4
  Out04 : Outport  Port=5
  Out10 : Outport  Port=6
  Out11 : Outport  Port=7
  Out12 : Outport  Port=8
  Out13 : Outport  Port=9
  Out14 : Outport  Port=10
  Out20 : Outport  Port=11
  Out21 : Outport  Port=12
  Out22 : Outport  Port=13
  Out23 : Outport  Port=14
  Out24 : Outport  Port=15
  Out30 : Outport  Port=16
  Out31 : Outport  Port=17
  Out32 : Outport  Port=18
  Out33 : Outport  Port=19
  Out34 : Outport  Port=20
  Out40 : Outport  Port=21
  Out41 : Outport  Port=22
  Out42 : Outport  Port=23
  Out43 : Outport  Port=24
  Out44 : Outport  Port=25
  wires:
  [clken] -> Delay11/2
  Delay11/1 -> [data_23], Delay12/1
  [clken] -> Delay12/2
  [clken] -> Delay10/2
  Delay8/1 -> Memory Delay1/1, [data_14]
  [clken] -> Memory Delay1/2
  Delay9/1 -> [data_21], Delay10/1
  Memory Delay1/1 -> [data_20], Delay9/1
  Delay10/1 -> [data_22], Delay11/1
  [clken] -> Delay9/2
  [clken] -> Delay4/2
  [data_03] -> Out03/1
  [data_04] -> Out04/1
  [data_02] -> Out02/1
  Delay/1 -> [data_00], Delay1/1
  [data_32] -> Out32/1
  [data_44] -> Out44/1
  [data_31] -> Out31/1
  [data_40] -> Out40/1
  [data_34] -> Out34/1
  [data_30] -> Out30/1
  [data_33] -> Out33/1
  [data_43] -> Out43/1
  [data_42] -> Out42/1
  [data_41] -> Out41/1
  [clken] -> Delay1/2
  [clken] -> Delay/2
  [data_in] -> Delay/1
  [clken] -> Delay2/2
  Delay2/1 -> [data_02], Delay3/1
  Delay1/1 -> [data_01], Delay2/1
  [clken] -> Delay3/2
  [data_01] -> Out01/1
  clken/1 -> [clken]
  [data_00] -> Out00/1
  [data_21] -> Out21/1
  [data_20] -> Out20/1
  [data_23] -> Out23/1
  [data_22] -> Out22/1
  [data_24] -> Out24/1
  dataIn/1 -> [data_in]
  [data_10] -> Out10/1
  [data_11] -> Out11/1
  [data_12] -> Out12/1
  [data_13] -> Out13/1
  [data_14] -> Out14/1
  Delay4/1 -> Memory Delay/1, [data_04]
  [clken] -> Memory Delay/2
  Delay12/1 -> [data_24], Memory Delay2/1
  [clken] -> Memory Delay2/2
  Memory Delay2/1 -> [data_30], Delay16/1
  [clken] -> Delay16/2
  [clken] -> Delay14/2
  [clken] -> Delay15/2
  [clken] -> Memory Delay3/2
  Delay17/1 -> [data_32], Delay18/1
  Delay18/1 -> [data_33], Delay19/1
  Memory Delay3/1 -> [data_40], Delay20/1
  [clken] -> Delay20/2
  [clken] -> Delay19/2
  Delay13/1 -> [data_42], Delay14/1
  Delay19/1 -> Memory Delay3/1, [data_34]
  Delay14/1 -> [data_43], Delay15/1
  Delay15/1 -> [data_44]
  [clken] -> Delay17/2
  [clken] -> Delay18/2
  [clken] -> Delay13/2
  Delay16/1 -> [data_31], Delay17/1
  Delay20/1 -> [data_41], Delay13/1
  Memory Delay/1 -> [data_10], Delay5/1
  [clken] -> Delay7/2
  [clken] -> Delay6/2
  Delay5/1 -> [data_11], Delay6/1
  [clken] -> Delay8/2
  [clken] -> Delay5/2
  Delay7/1 -> [data_13], Delay8/1
  Delay6/1 -> [data_12], Delay7/1
  Delay3/1 -> [data_03], Delay4/1
